simulink model "HoppingModel_Last"  (R2019b)
settings: Solver=FixedStepAuto  StartTime=0.0  StopTime=20  FixedStep=0.005  RelTol=1e-3
undefined symbols (not defined in the file): g, I1, I2, ini_theta1, ini_theta1_d, ini_theta2, ini_theta2_d, ini_w, ini_w_d, ini_x0, ini_x0_d, ini_x1, ini_x1_d, ini_x2, ini_x2_d, ini_y0, ini_y0_d, ini_y1, ini_y1_d, ini_y2, ini_y2_d, M1, M2, r1, r2, theta1_des
libraries: cstblocks x5
settings Model: Creator=fabia  LastModifiedBy=fabia

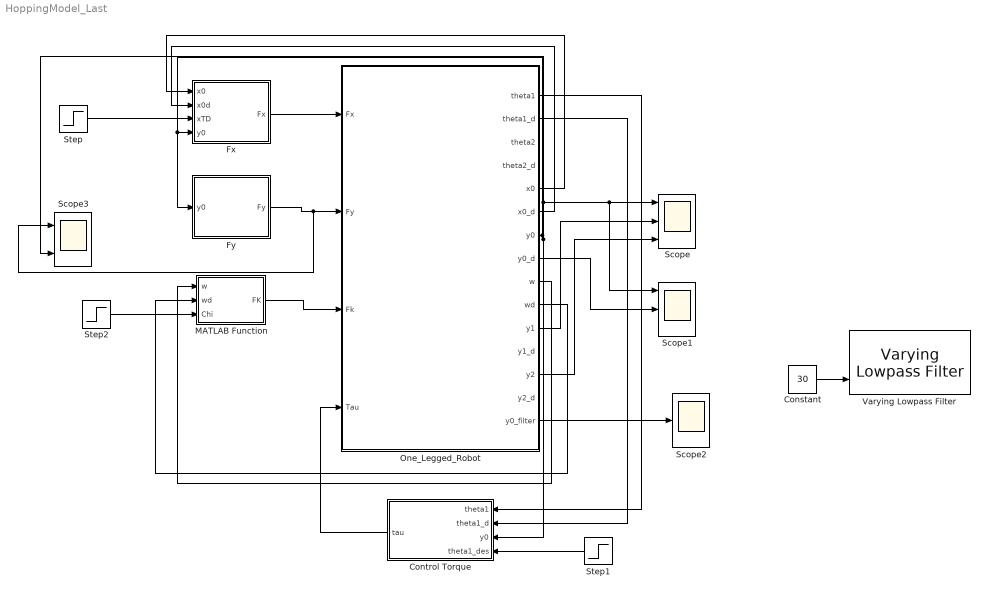
== system HoppingModel_Last ==
  Constant : Constant  Value=30
  Control Torque : MATLAB Function  TreatAsAtomicUnit=on
  Fx : MATLAB Function  TreatAsAtomicUnit=on
  Fy : MATLAB Function  TreatAsAtomicUnit=on
  MATLAB Function : MATLAB Function  TreatAsAtomicUnit=on
  One_Legged_Robot : Subsystem
  Scope : Scope  NumInputPorts=3
  Scope1 : Scope  NumInputPorts=3
  Scope2 : Scope
  Scope3 : Scope  NumInputPorts=2
  Step : Step  Time=0  After=0  SampleTime=0
  Step1 : Step  Time=0  After=theta1_des  SampleTime=0
  Step2 : Step  Time=0  After=0.1  SampleTime=0
  Varying Lowpass Filter : cstblocks/Linear Parameter Varying/Varying Lowpass Filter  N=1
      settings: SourceProductName=Control System Toolbox
  wires:
  Fx/1(Fx) -> One_Legged_Robot/1(Fx)
  One_Legged_Robot/6(x0_d) -> Fx/2(x0d)
  Step/1 -> Fx/3(xTD)
  Step2/1 -> MATLAB Function/3(Chi)
  Control Torque/1(tau) -> One_Legged_Robot/4(Tau)
  One_Legged_Robot/1(theta1) -> Control Torque/1(theta1)
  One_Legged_Robot/2(theta1_d) -> Control Torque/2(theta1_d)
  Step1/1 -> Control Torque/4(theta1_des)
  One_Legged_Robot/11(y1) -> Scope/2
  One_Legged_Robot/13(y2) -> Scope/3
  One_Legged_Robot/7(y0) -> Fy/1(y0), Fx/4(y0), Scope3/2, Scope1/1, Scope/1, Control Torque/3(y0)
  Constant/1 -> Varying Lowpass Filter/2
  One_Legged_Robot/5(x0) -> Fx/1(x0)
  Fy/1(Fy) -> Scope3/1, One_Legged_Robot/2(Fy)
  One_Legged_Robot/9(w) -> MATLAB Function/1(w)
  One_Legged_Robot/10(wd) -> MATLAB Function/2(wd)
  One_Legged_Robot/8(y0_d) -> Scope1/2
  One_Legged_Robot/15(y0_filter) -> Scope2/1
  MATLAB Function/1(FK) -> One_Legged_Robot/3(Fk)

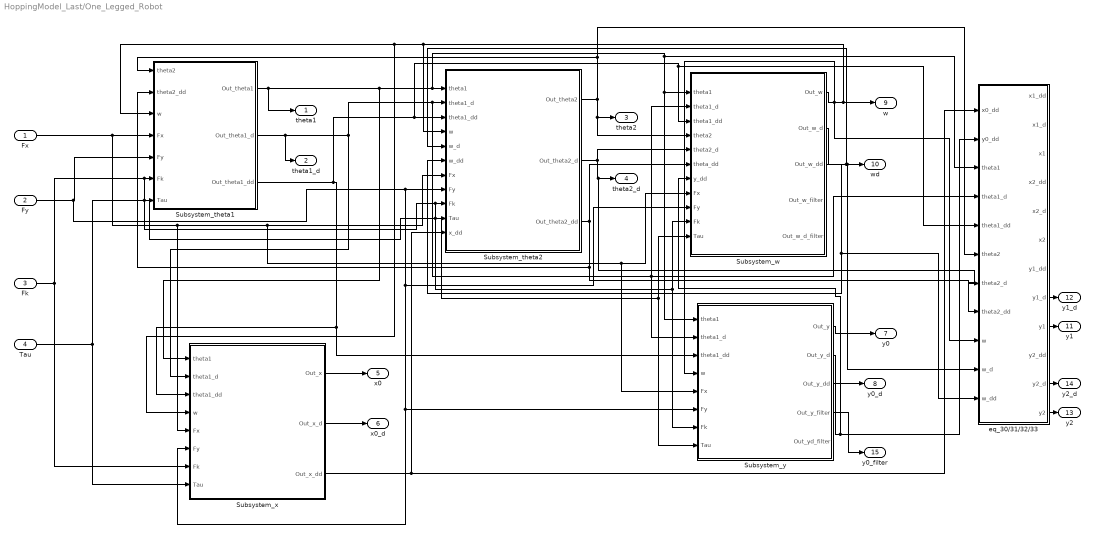
== system HoppingModel_Last/One_Legged_Robot ==
  Fx : Inport
  Fy : Inport  Port=2
  Fk : Inport  Port=3
  Tau : Inport  Port=4
  Subsystem_theta1 : Subsystem
  Subsystem_theta2 : Subsystem
  Subsystem_w : Subsystem
  Subsystem_x : Subsystem
  Subsystem_y : Subsystem
  "eq_30/31/32/33 " : Subsystem
  theta1 : Outport
  theta1_d : Outport  Port=2
  theta2 : Outport  Port=3
  theta2_d : Outport  Port=4
  x0 : Outport  Port=5
  x0_d : Outport  Port=6
  y0 : Outport  Port=7
  y0_d : Outport  Port=8
  w : Outport  Port=9
  wd : Outport  Port=10
  y1 : Outport  Port=11
  y1_d : Outport  Port=12
  y2 : Outport  Port=13
  y2_d : Outport  Port=14
  y0_filter : Outport  Port=15
  wires:
  Subsystem_theta1/1(Out_theta1) -> Subsystem_x/1(theta1), "eq_30/31/32/33 "/3(theta1), Subsystem_y/1(theta1), Subsystem_w/1(theta1), Subsystem_theta2/1(theta1), theta1/1
  Subsystem_theta1/2(Out_theta1_d) -> Subsystem_y/2(theta1_d), "eq_30/31/32/33 "/4(theta1_d), Subsystem_w/2(theta1_d), Subsystem_theta2/2(theta1_d), Subsystem_x/2(theta1_d), theta1_d/1
  Subsystem_x/1(Out_x) -> x0/1
  Subsystem_x/2(Out_x_d) -> x0_d/1
  Subsystem_y/1(Out_y) -> y0/1
  Subsystem_y/2(Out_y_d) -> y0_d/1
  "eq_30/31/32/33 "/9(y1) -> y1/1
  "eq_30/31/32/33 "/8(y1_d) -> y1_d/1
  "eq_30/31/32/33 "/12(y2) -> y2/1
  "eq_30/31/32/33 "/11(y2_d) -> y2_d/1
  Subsystem_w/2(Out_w_d) -> "eq_30/31/32/33 "/10(w_d), wd/1, Subsystem_theta2/5(w_d)
  Subsystem_w/1(Out_w) -> Subsystem_y/4(w), "eq_30/31/32/33 "/9(w), Subsystem_theta2/4(w), Subsystem_x/4(w), Subsystem_theta1/3(w), w/1
  Subsystem_theta2/1(Out_theta2) -> "eq_30/31/32/33 "/6(theta2), Subsystem_theta1/1(theta2), Subsystem_w/4(theta2), theta2/1
  Subsystem_theta2/2(Out_theta2_d) -> Subsystem_w/5(theta2_d), "eq_30/31/32/33 "/7(theta2_d), theta2_d/1
  Subsystem_theta1/3(Out_theta1_dd) -> Subsystem_x/3(theta1_dd), Subsystem_y/3(theta1_dd), "eq_30/31/32/33 "/5(theta1_dd), Subsystem_w/3(theta1_dd), Subsystem_theta2/3(theta1_dd)
  Subsystem_theta2/3(Out_theta2_dd) -> "eq_30/31/32/33 "/8(theta2_dd), Subsystem_theta1/2(theta2_dd), Subsystem_w/6(theta_dd)
  Subsystem_w/3(Out_w_dd) -> "eq_30/31/32/33 "/11(w_dd), Subsystem_theta2/6(w_dd)
  Subsystem_y/3(Out_y_dd) -> "eq_30/31/32/33 "/2(y0_dd), Subsystem_w/7(y_dd)
  Subsystem_x/3(Out_x_dd) -> "eq_30/31/32/33 "/1(x0_dd), Subsystem_theta2/11(x_dd)
  Fx/1 -> Subsystem_x/5(Fx), Subsystem_y/5(Fx), Subsystem_w/8(Fx), Subsystem_theta2/7(Fx), Subsystem_theta1/4(Fx)
  Fy/1 -> Subsystem_w/9(Fy), Subsystem_x/6(Fy), Subsystem_y/6(Fy), Subsystem_theta2/8(Fy), Subsystem_theta1/5(Fy)
  Fk/1 -> Subsystem_x/7(Fk), Subsystem_y/7(Fk), Subsystem_w/10(Fk), Subsystem_theta2/9(Fk), Subsystem_theta1/6(Fk)
  Tau/1 -> Subsystem_x/8(Tau), Subsystem_y/8(Tau), Subsystem_w/11(Tau), Subsystem_theta2/10(Tau), Subsystem_theta1/7(Tau)
  Subsystem_y/4(Out_y_filter) -> y0_filter/1

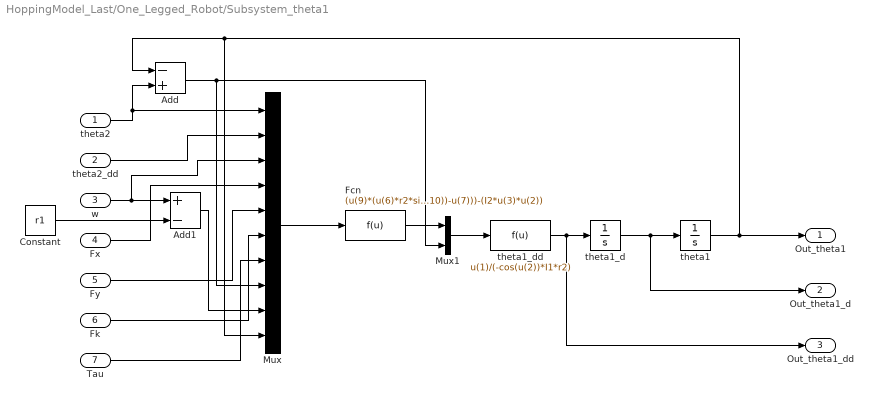
== system HoppingModel_Last/One_Legged_Robot/Subsystem_theta1 ==
  theta2 : Inport
  theta2_dd : Inport  Port=2
  w : Inport  Port=3
  Fx : Inport  Port=4
  Fy : Inport  Port=5
  Fk : Inport  Port=6
  Tau : Inport  Port=7
  Add : Sum  Inputs=-+
  Add1 : Sum  Inputs=+-
  Constant : Constant  Value=r1
  Fcn : Fcn  Expr=(u(9)*(u(6)*r2*sin(u(8))+u(7)))-(r2*cos(u(8))*(r1*u(5)*sin(u(10))-r1*u(4)*cos(u(10))-u(7)))-(I2*u(3)*u(2))
  Mux : Mux  Inputs=10
  Mux1 : Mux  Inputs=2
  theta1 : Integrator  InitialCondition=ini_theta1  LimitOutput=on  UpperSaturationLimit=pi/2  LowerSaturationLimit=-pi/2
  theta1_d : Integrator  InitialCondition=ini_theta1_d  LimitOutput=on  UpperSaturationLimit=pi/2  LowerSaturationLimit=-pi/2
  theta1_dd : Fcn  Expr=u(1)/(-cos(u(2))*I1*r2)
  Out_theta1 : Outport
  Out_theta1_d : Outport  Port=2
  Out_theta1_dd : Outport  Port=3
  wires:
  theta2/1 -> Mux/1, Add/2
  theta1/1 -> Out_theta1/1, Mux/10, Add/1
  w/1 -> Mux/3, Add1/1
  Constant/1 -> Add1/2
  theta2_dd/1 -> Mux/2
  Fx/1 -> Mux/4
  Fy/1 -> Mux/5
  Fk/1 -> Mux/6
  Tau/1 -> Mux/7
  Add/1 -> Mux/8, Mux1/2
  Add1/1 -> Mux/9
  Mux/1 -> Fcn/1
  Fcn/1 -> Mux1/1
  Mux1/1 -> theta1_dd/1
  theta1_dd/1 -> Out_theta1_dd/1, theta1_d/1
  theta1_d/1 -> Out_theta1_d/1, theta1/1

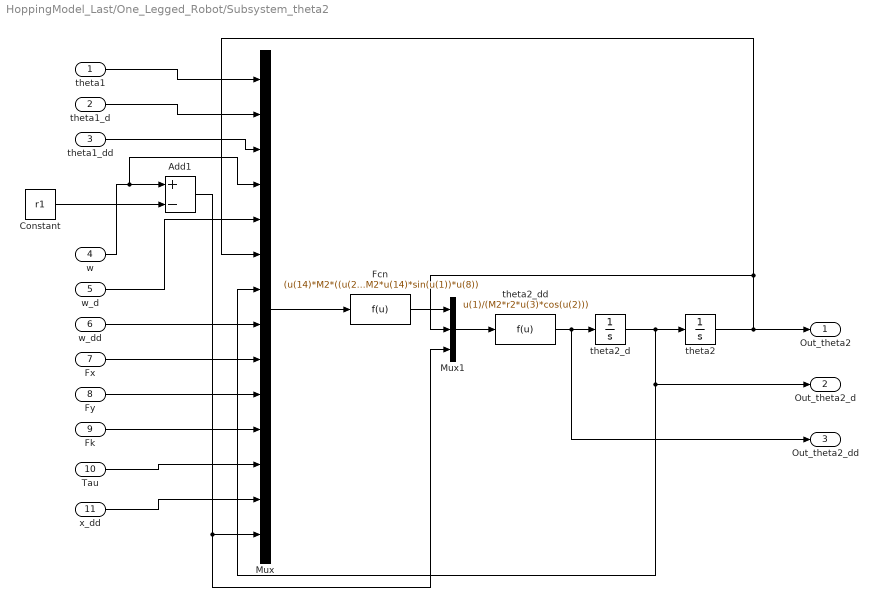
== system HoppingModel_Last/One_Legged_Robot/Subsystem_theta2 ==
  theta1 : Inport
  theta1_d : Inport  Port=2
  theta1_dd : Inport  Port=3
  w : Inport  Port=4
  w_d : Inport  Port=5
  w_dd : Inport  Port=6
  Fx : Inport  Port=7
  Fy : Inport  Port=8
  Fk : Inport  Port=9
  Tau : Inport  Port=10
  x_dd : Inport  Port=11
  Add1 : Sum  Inputs=+-
  Constant : Constant  Value=r1
  Fcn : Fcn  Expr=(u(14)*M2*((u(2)^2)*u(14)*sin(u(1))-2*u(2)*u(5)*cos(u(1))+r2*(u(7)^2)*sin(u(6))+r1*(u(2)^2)*sin(u(1))))-(r1*u(9)*(cos(u(1)))^2)+(cos(u(1))*(r1*u(10)*sin(u(1))-u(12)))+(u(11)*u(14)*sin(u(1)))-(M2*u(14)*u(13))-(cos(u(1))*(M2*u(14)*u(4)+I1)*u(3))-(M2*u(14)*sin(u(1))*u(8))
  Mux : Mux  Inputs=14
  Mux1 : Mux  Inputs=3
  theta2 : Integrator  InitialCondition=ini_theta2
  theta2_d : Integrator  InitialCondition=ini_theta2_d
  theta2_dd : Fcn  Expr=u(1)/(M2*r2*u(3)*cos(u(2)))
  Out_theta2 : Outport
  Out_theta2_d : Outport  Port=2
  Out_theta2_dd : Outport  Port=3
  wires:
  theta2/1 -> Mux1/2, Mux/6, Out_theta2/1
  Fcn/1 -> Mux1/1
  Mux1/1 -> theta2_dd/1
  theta2_dd/1 -> Out_theta2_dd/1, theta2_d/1
  theta2_d/1 -> Mux/7, Out_theta2_d/1, theta2/1
  Constant/1 -> Add1/2
  theta1/1 -> Mux/1
  theta1_d/1 -> Mux/2
  theta1_dd/1 -> Mux/3
  Add1/1 -> Mux1/3, Mux/14
  Mux/1 -> Fcn/1
  w/1 -> Mux/4, Add1/1
  w_d/1 -> Mux/5
  w_dd/1 -> Mux/8
  Fx/1 -> Mux/9
  Fy/1 -> Mux/10
  Fk/1 -> Mux/11
  Tau/1 -> Mux/12
  x_dd/1 -> Mux/13

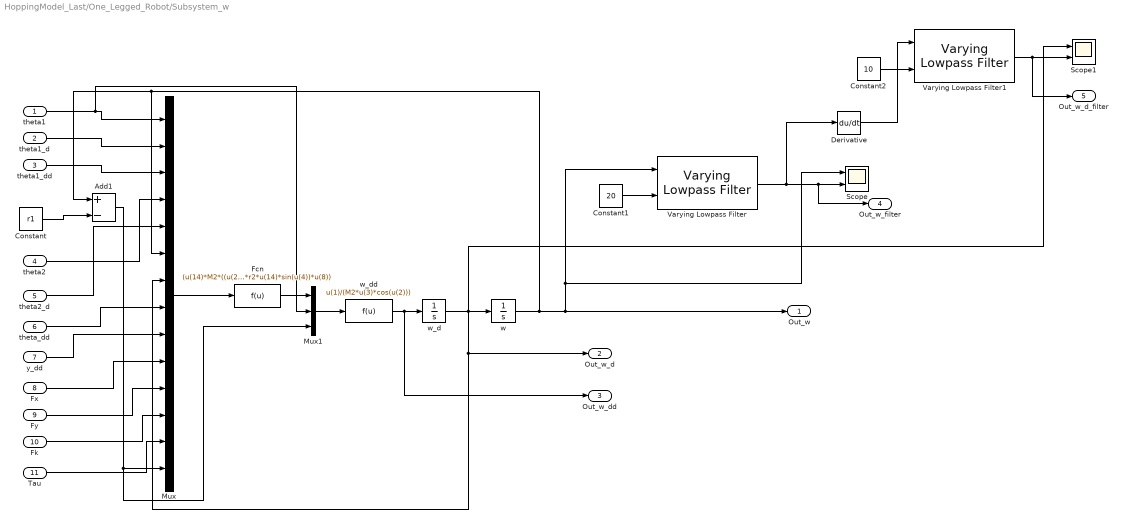
== system HoppingModel_Last/One_Legged_Robot/Subsystem_w ==
  theta1 : Inport
  theta1_d : Inport  Port=2
  theta1_dd : Inport  Port=3
  theta2 : Inport  Port=4
  theta2_d : Inport  Port=5
  theta_dd : Inport  Port=6
  y_dd : Inport  Port=7
  Fx : Inport  Port=8
  Fy : Inport  Port=9
  Fk : Inport  Port=10
  Tau : Inport  Port=11
  Add1 : Sum  Inputs=+-
  Constant : Constant  Value=r1
  Constant1 : Constant  Value=20
  Constant2 : Constant  Value=10
  Derivative : Derivative
  Fcn : Fcn  Expr=(u(14)*M2*((u(2)^2)*u(14)*cos(u(1))+2*u(2)*u(7)*sin(u(1))+r2*(u(5)^2)*cos(u(4))+r1*(u(2)^2)*cos(u(1))-g))+(r1*u(10)*cos(u(1))*sin(u(1)))-(sin(u(1))*(r1*u(11)*sin(u(1))-u(13)))+(u(12)*u(14)*cos(u(1)))+(sin(u(1))*(M2*u(14)*u(6)+I1)*u(3))-(M2*u(14)*u(9))+(M2*r2*u(14)*sin(u(4))*u(8))
  Mux : Mux  Inputs=14
  Mux1 : Mux  Inputs=3
  Scope : Scope  NumInputPorts=2
  Scope1 : Scope  NumInputPorts=2
  Varying Lowpass Filter : cstblocks/Linear Parameter Varying/Varying Lowpass Filter  N=1
      settings: SourceProductName=Control System Toolbox
  Varying Lowpass Filter1 : cstblocks/Linear Parameter Varying/Varying Lowpass Filter  N=1
      settings: SourceProductName=Control System Toolbox
  w : Integrator  InitialCondition=ini_w
  w_d : Integrator  InitialCondition=ini_w_d
  w_dd : Fcn  Expr=u(1)/(M2*u(3)*cos(u(2)))
  Out_w : Outport
  Out_w_d : Outport  Port=2
  Out_w_dd : Outport  Port=3
  Out_w_filter : Outport  Port=4
  Out_w_d_filter : Outport  Port=5
  wires:
  Fcn/1 -> Mux1/1
  Mux1/1 -> w_dd/1
  w_dd/1 -> Out_w_dd/1, w_d/1
  w_d/1 -> Scope1/1, Mux/7, Out_w_d/1, w/1
  Constant/1 -> Add1/2
  Mux/1 -> Fcn/1
  Add1/1 -> Mux1/3, Mux/14
  theta1/1 -> Mux1/2, Mux/1
  theta1_d/1 -> Mux/2
  theta1_dd/1 -> Mux/3
  theta2/1 -> Mux/4
  theta2_d/1 -> Mux/5
  theta_dd/1 -> Mux/8
  y_dd/1 -> Mux/9
  Fx/1 -> Mux/10
  Fy/1 -> Mux/11
  Fk/1 -> Mux/12
  Tau/1 -> Mux/13
  Constant1/1 -> Varying Lowpass Filter/2
  w/1 -> Mux/6, Add1/1, Out_w/1, Scope/1, Varying Lowpass Filter/1
  Derivative/1 -> Varying Lowpass Filter1/1
  Constant2/1 -> Varying Lowpass Filter1/2
  Varying Lowpass Filter/1 -> Derivative/1, Out_w_filter/1, Scope/2
  Varying Lowpass Filter1/1 -> Out_w_d_filter/1, Scope1/2

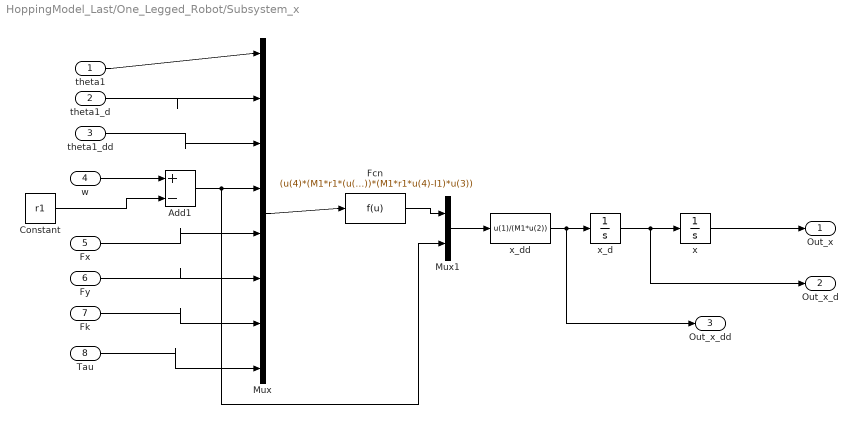
== system HoppingModel_Last/One_Legged_Robot/Subsystem_x ==
  theta1 : Inport
  theta1_d : Inport  Port=2
  theta1_dd : Inport  Port=3
  w : Inport  Port=4
  Fx : Inport  Port=5
  Fy : Inport  Port=6
  Fk : Inport  Port=7
  Tau : Inport  Port=8
  Add1 : Sum  Inputs=+-
  Constant : Constant  Value=r1
  Fcn : Fcn  Expr=(u(4)*(M1*r1*(u(2)^2)*sin(u(1))-u(7)*sin(u(1))+u(5)))-(cos(u(1))*(u(6)*r1*sin(u(1))-u(5)*r1*cos(u(1))-u(8)))-(cos(u(1))*(M1*r1*u(4)-I1)*u(3))
  Mux : Mux  Inputs=8
  Mux1 : Mux  Inputs=2
  x : Integrator  InitialCondition=ini_x0
  x_d : Integrator  InitialCondition=ini_x0_d
  x_dd : Fcn  Expr=u(1)/(M1*u(2))
  Out_x : Outport
  Out_x_d : Outport  Port=2
  Out_x_dd : Outport  Port=3
  wires:
  x/1 -> Out_x/1
  Fcn/1 -> Mux1/1
  Mux1/1 -> x_dd/1
  x_dd/1 -> Out_x_dd/1, x_d/1
  x_d/1 -> Out_x_d/1, x/1
  Constant/1 -> Add1/2
  Mux/1 -> Fcn/1
  w/1 -> Add1/1
  theta1/1 -> Mux/1
  theta1_d/1 -> Mux/2
  theta1_dd/1 -> Mux/3
  Add1/1 -> Mux1/2, Mux/4
  Fx/1 -> Mux/5
  Fy/1 -> Mux/6
  Fk/1 -> Mux/7
  Tau/1 -> Mux/8

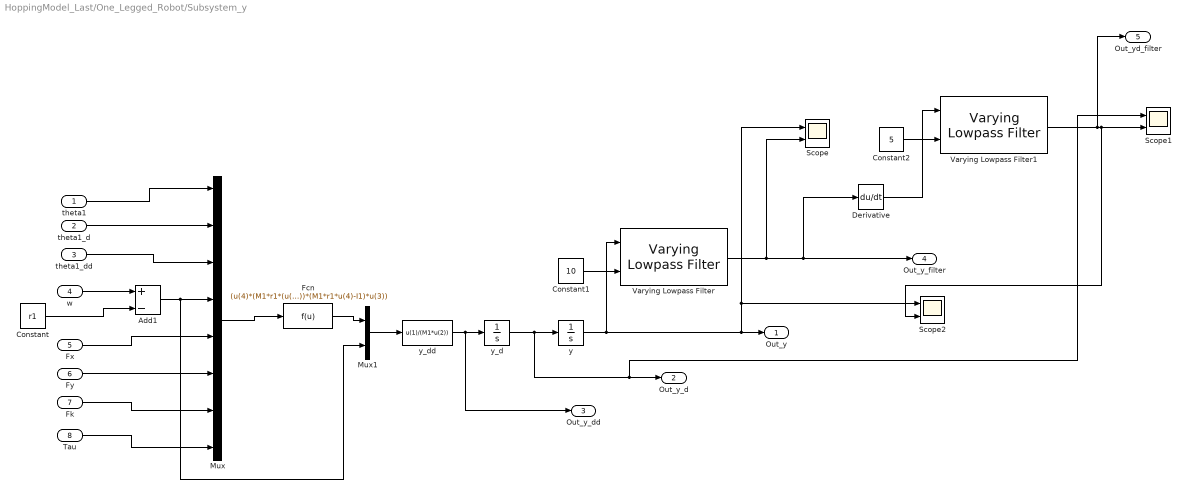
== system HoppingModel_Last/One_Legged_Robot/Subsystem_y ==
  theta1 : Inport
  theta1_d : Inport  Port=2
  theta1_dd : Inport  Port=3
  w : Inport  Port=4
  Fx : Inport  Port=5
  Fy : Inport  Port=6
  Fk : Inport  Port=7
  Tau : Inport  Port=8
  Add1 : Sum  Inputs=+-
  Constant : Constant  Value=r1
  Constant1 : Constant  Value=10
  Constant2 : Constant  Value=5
  Derivative : Derivative
  Fcn : Fcn  Expr=(u(4)*(M1*r1*(u(2)^2)*cos(u(1))-u(7)*cos(u(1))+u(6)-M1*g))-(sin(u(1))*(u(6)*r1*sin(u(1))-u(5)*r1*cos(u(1))-u(8)))+(sin(u(1))*(M1*r1*u(4)-I1)*u(3))
  Mux : Mux  Inputs=8
  Mux1 : Mux  Inputs=2
  Scope : Scope  NumInputPorts=2
  Scope1 : Scope  NumInputPorts=2
  Scope2 : Scope  NumInputPorts=2
  Varying Lowpass Filter : cstblocks/Linear Parameter Varying/Varying Lowpass Filter  N=1
      settings: SourceProductName=Control System Toolbox
  Varying Lowpass Filter1 : cstblocks/Linear Parameter Varying/Varying Lowpass Filter  N=1
      settings: SourceProductName=Control System Toolbox
  y : Integrator  InitialCondition=ini_y0
  y_d : Integrator  InitialCondition=ini_y0_d
  y_dd : Fcn  Expr=u(1)/(M1*u(2))
  Out_y : Outport
  Out_y_d : Outport  Port=2
  Out_y_dd : Outport  Port=3
  Out_y_filter : Outport  Port=4
  Out_yd_filter : Outport  Port=5
  wires:
  Fcn/1 -> Mux1/1
  Mux1/1 -> y_dd/1
  y_dd/1 -> Out_y_dd/1, y_d/1
  y_d/1 -> Scope1/1, Out_y_d/1, y/1
  Constant/1 -> Add1/2
  Mux/1 -> Fcn/1
  w/1 -> Add1/1
  theta1/1 -> Mux/1
  theta1_d/1 -> Mux/2
  theta1_dd/1 -> Mux/3
  Add1/1 -> Mux1/2, Mux/4
  Fx/1 -> Mux/5
  Fy/1 -> Mux/6
  Fk/1 -> Mux/7
  Tau/1 -> Mux/8
  Constant1/1 -> Varying Lowpass Filter/2
  Varying Lowpass Filter/1 -> Derivative/1, Out_y_filter/1, Scope/2
  Constant2/1 -> Varying Lowpass Filter1/2
  Derivative/1 -> Varying Lowpass Filter1/1
  Varying Lowpass Filter1/1 -> Scope1/2, Scope2/2, Out_yd_filter/1
  y/1 -> Scope2/1, Scope/1, Out_y/1, Varying Lowpass Filter/1

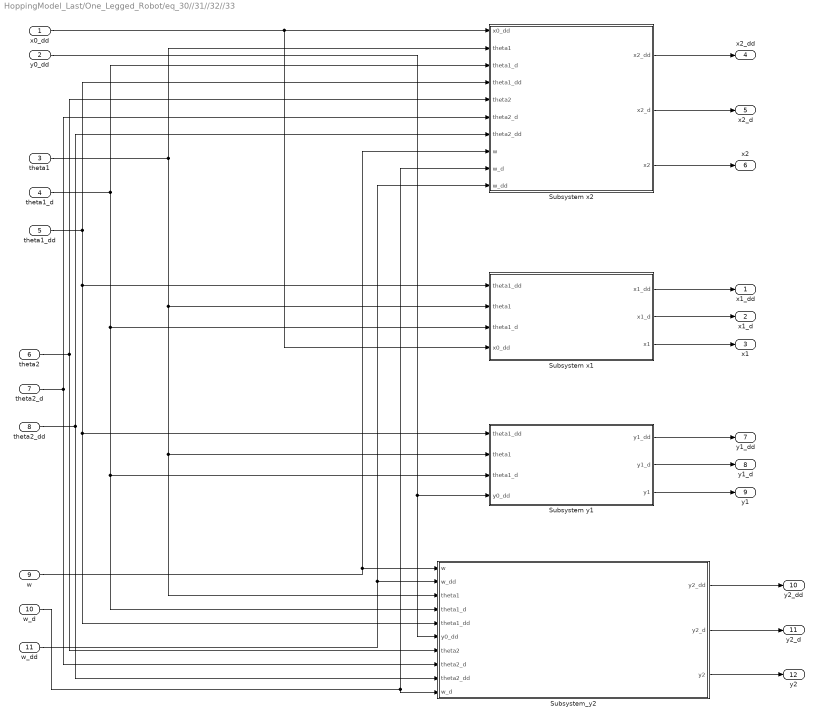
== system HoppingModel_Last/One_Legged_Robot/eq_30//31//32//33  ==
  x0_dd : Inport
  y0_dd : Inport  Port=2
  theta1 : Inport  Port=3
  theta1_d : Inport  Port=4
  theta1_dd : Inport  Port=5
  theta2 : Inport  Port=6
  theta2_d : Inport  Port=7
  theta2_dd : Inport  Port=8
  w : Inport  Port=9
  w_d : Inport  Port=10
  w_dd : Inport  Port=11
  Subsystem x1 : Subsystem
  Subsystem x2 : Subsystem
  Subsystem y1 : Subsystem
  Subsystem_y2 : Subsystem
  x1_dd : Outport
  x1_d : Outport  Port=2
  x1 : Outport  Port=3
  x2_dd : Outport  Port=4
  x2_d : Outport  Port=5
  x2 : Outport  Port=6
  y1_dd : Outport  Port=7
  y1_d : Outport  Port=8
  y1 : Outport  Port=9
  y2_dd : Outport  Port=10
  y2_d : Outport  Port=11
  y2 : Outport  Port=12
  wires:
  Subsystem x1/1(x1_dd) -> x1_dd/1
  Subsystem x1/3(x1) -> x1/1
  x0_dd/1 -> Subsystem x1/4(x0_dd), Subsystem x2/1(x0_dd)
  Subsystem_y2/1(y2_dd) -> y2_dd/1
  theta1_d/1 -> Subsystem_y2/4(theta1_d), Subsystem y1/3(theta1_d), Subsystem x1/3(theta1_d), Subsystem x2/3(theta1_d)
  Subsystem x2/1(x2_dd) -> x2_dd/1
  Subsystem x2/3(x2) -> x2/1
  w_dd/1 -> Subsystem x2/10(w_dd), Subsystem_y2/2(w_dd)
  Subsystem_y2/3(y2) -> y2/1
  theta1/1 -> Subsystem_y2/3(theta1), Subsystem y1/2(theta1), Subsystem x1/2(theta1), Subsystem x2/2(theta1)
  Subsystem x1/2(x1_d) -> x1_d/1
  theta1_dd/1 -> Subsystem_y2/5(theta1_dd), Subsystem y1/1("theta1_dd "), Subsystem x1/1("theta1_dd "), Subsystem x2/4(theta1_dd)
  y0_dd/1 -> Subsystem_y2/6(y0_dd), Subsystem y1/4(y0_dd)
  theta2_dd/1 -> Subsystem x2/7("theta2_dd "), Subsystem_y2/9(theta2_dd)
  w_d/1 -> Subsystem_y2/10(w_d), Subsystem x2/9(w_d)
  Subsystem x2/2(x2_d) -> x2_d/1
  Subsystem y1/3(y1) -> y1/1
  theta2_d/1 -> Subsystem x2/6(theta2_d), Subsystem_y2/8(theta2_d)
  theta2/1 -> Subsystem x2/5(theta2), Subsystem_y2/7(theta2)
  w/1 -> Subsystem x2/8(w), Subsystem_y2/1(w)
  Subsystem y1/2(y1_d) -> y1_d/1
  Subsystem y1/1(y1_dd) -> y1_dd/1
  Subsystem_y2/2(y2_d) -> y2_d/1

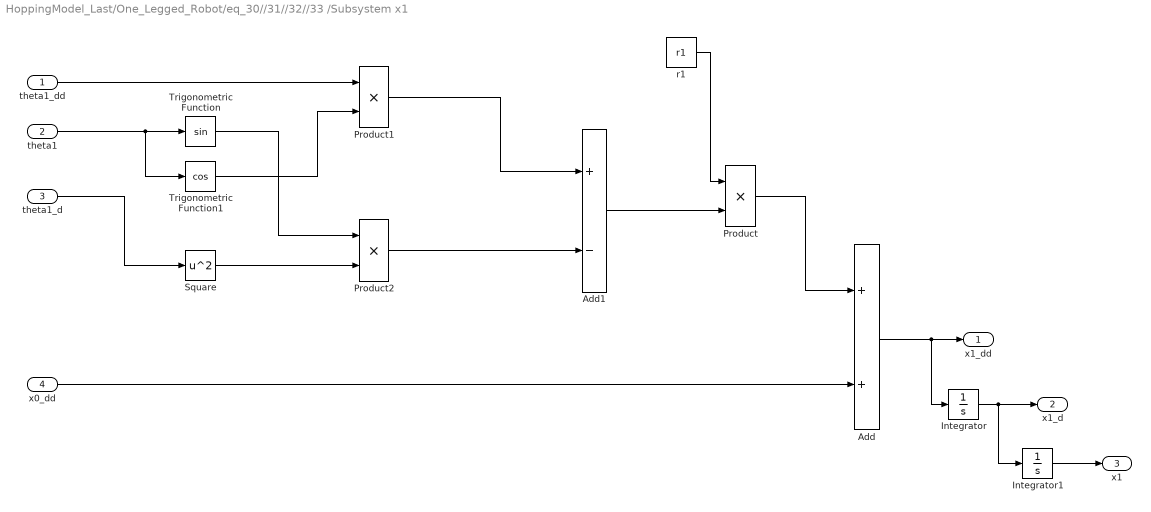
== system HoppingModel_Last/One_Legged_Robot/eq_30//31//32//33 /Subsystem x1 ==
  "theta1_dd " : Inport
  theta1 : Inport  Port=2
  theta1_d : Inport  Port=3
  x0_dd : Inport  Port=4
  Add : Sum
  Add1 : Sum  Inputs=+-
  Integrator : Integrator  InitialCondition=ini_x1_d
  Integrator1 : Integrator  InitialCondition=ini_x1
  Product : Product
  Product1 : Product
  Product2 : Product
  Square : Math  Operator=square  SignedPower=off  SaturateOnIntegerOverflow=on
  Trigonometric Function : Trigonometry
  Trigonometric Function1 : Trigonometry  Operator=cos
  r1 : Constant  Value=r1
  x1_dd : Outport
  x1_d : Outport  Port=2
  x1 : Outport  Port=3
  wires:
  Add1/1 -> Product/2
  Product/1 -> Add/1
  Product2/1 -> Add1/2
  r1/1 -> Product/1
  Trigonometric Function1/1 -> Product1/2
  x0_dd/1 -> Add/2
  theta1_d/1 -> Square/1
  Trigonometric Function/1 -> Product2/1
  Integrator/1 -> x1_d/1, Integrator1/1
  Add/1 -> x1_dd/1, Integrator/1
  Square/1 -> Product2/2
  Product1/1 -> Add1/1
  "theta1_dd "/1 -> Product1/1
  theta1/1 -> Trigonometric Function1/1, Trigonometric Function/1
  Integrator1/1 -> x1/1

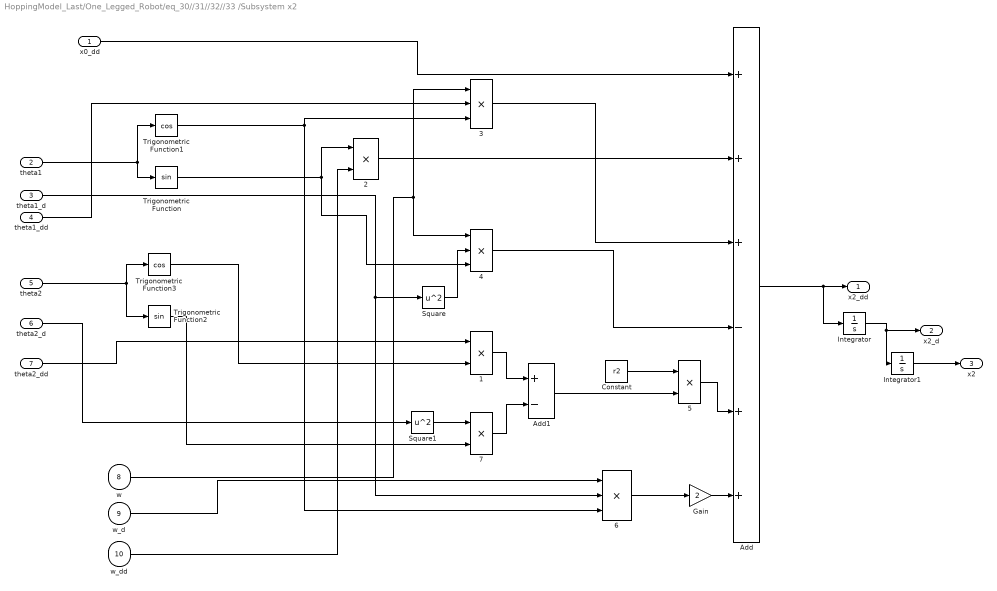
== system HoppingModel_Last/One_Legged_Robot/eq_30//31//32//33 /Subsystem x2 ==
  x0_dd : Inport
  theta1 : Inport  Port=2
  theta1_d : Inport  Port=3
  theta1_dd : Inport  Port=4
  theta2 : Inport  Port=5
  theta2_d : Inport  Port=6
  "theta2_dd " : Inport  Port=7
  w : Inport  Port=8
  w_d : Inport  Port=9
  w_dd : Inport  Port=10
  {1..2,5,7} (4 alike) : Product
  3 : Product  Inputs=3
  4 : Product  Inputs=3
  6 : Product  Inputs=3
  Add : Sum  Inputs=+++-++
  Add1 : Sum  Inputs=+-
  Constant : Constant  Value=r2
  Gain : Gain  Gain=2
  Integrator : Integrator  InitialCondition=ini_x2_d
  Integrator1 : Integrator  InitialCondition=ini_x2
  Square : Math  Operator=square  SignedPower=off  SaturateOnIntegerOverflow=on
  Square1 : Math  Operator=square  SignedPower=off  SaturateOnIntegerOverflow=on
  Trigonometric Function : Trigonometry
  Trigonometric Function1 : Trigonometry  Operator=cos
  Trigonometric Function2 : Trigonometry
  Trigonometric Function3 : Trigonometry  Operator=cos
  x2_dd : Outport
  x2_d : Outport  Port=2
  x2 : Outport  Port=3
  wires:
  7/1 -> Add1/2
  Integrator1/1 -> x2/1
  w_d/1 -> 6/1
  Constant/1 -> 5/1
  Integrator/1 -> x2_d/1, Integrator1/1
  Trigonometric Function1/1 -> 6/3, 3/3
  x0_dd/1 -> Add/1
  Add1/1 -> 5/2
  theta2/1 -> Trigonometric Function3/1, Trigonometric Function2/1
  6/1 -> Gain/1
  4/1 -> Add/4
  Square/1 -> 4/2
  theta1_d/1 -> 6/2, Square/1
  Square1/1 -> 7/1
  w/1 -> 3/1, 4/1
  Add/1 -> x2_dd/1, Integrator/1
  Trigonometric Function2/1 -> 7/2
  Trigonometric Function3/1 -> 1/2
  w_dd/1 -> 2/2
  theta1/1 -> Trigonometric Function1/1, Trigonometric Function/1
  Gain/1 -> Add/6
  Trigonometric Function/1 -> 4/3, 2/1
  theta1_dd/1 -> 3/2
  3/1 -> Add/3
  1/1 -> Add1/1
  2/1 -> Add/2
  5/1 -> Add/5
  "theta2_dd "/1 -> 1/1
  theta2_d/1 -> Square1/1

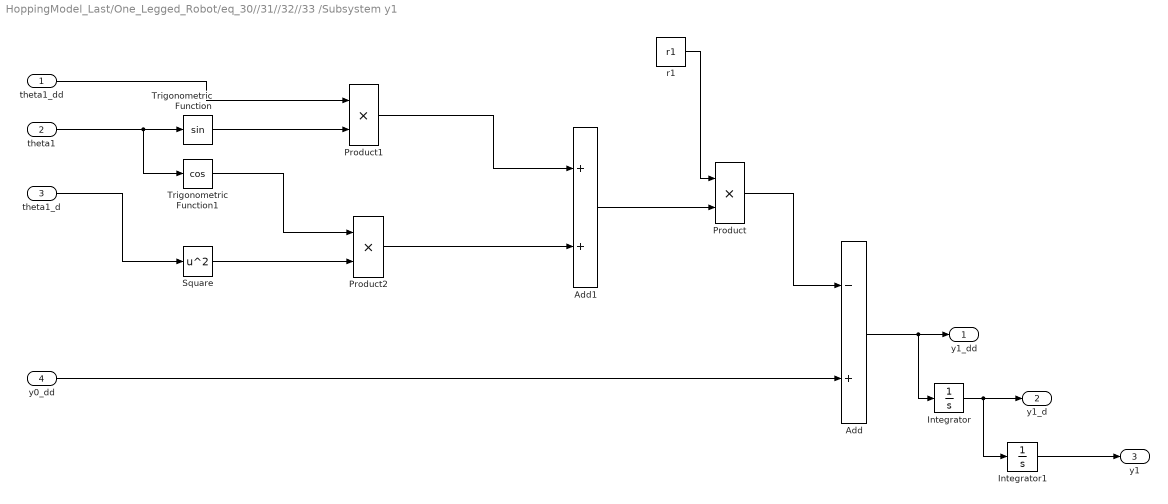
== system HoppingModel_Last/One_Legged_Robot/eq_30//31//32//33 /Subsystem y1 ==
  "theta1_dd " : Inport
  theta1 : Inport  Port=2
  theta1_d : Inport  Port=3
  y0_dd : Inport  Port=4
  Add : Sum  Inputs=-+
  Add1 : Sum
  Integrator : Integrator  InitialCondition=ini_y1_d
  Integrator1 : Integrator  InitialCondition=ini_y1
  Product : Product
  Product1 : Product
  Product2 : Product
  Square : Math  Operator=square  SignedPower=off  SaturateOnIntegerOverflow=on
  Trigonometric Function : Trigonometry
  Trigonometric Function1 : Trigonometry  Operator=cos
  r1 : Constant  Value=r1
  y1_dd : Outport
  y1_d : Outport  Port=2
  y1 : Outport  Port=3
  wires:
  "theta1_dd "/1 -> Product1/1
  Product1/1 -> Add1/1
  y0_dd/1 -> Add/2
  Integrator/1 -> y1_d/1, Integrator1/1
  Add/1 -> y1_dd/1, Integrator/1
  r1/1 -> Product/1
  Integrator1/1 -> y1/1
  theta1/1 -> Trigonometric Function1/1, Trigonometric Function/1
  Square/1 -> Product2/2
  theta1_d/1 -> Square/1
  Product/1 -> Add/1
  Trigonometric Function/1 -> Product1/2
  Product2/1 -> Add1/2
  Add1/1 -> Product/2
  Trigonometric Function1/1 -> Product2/1

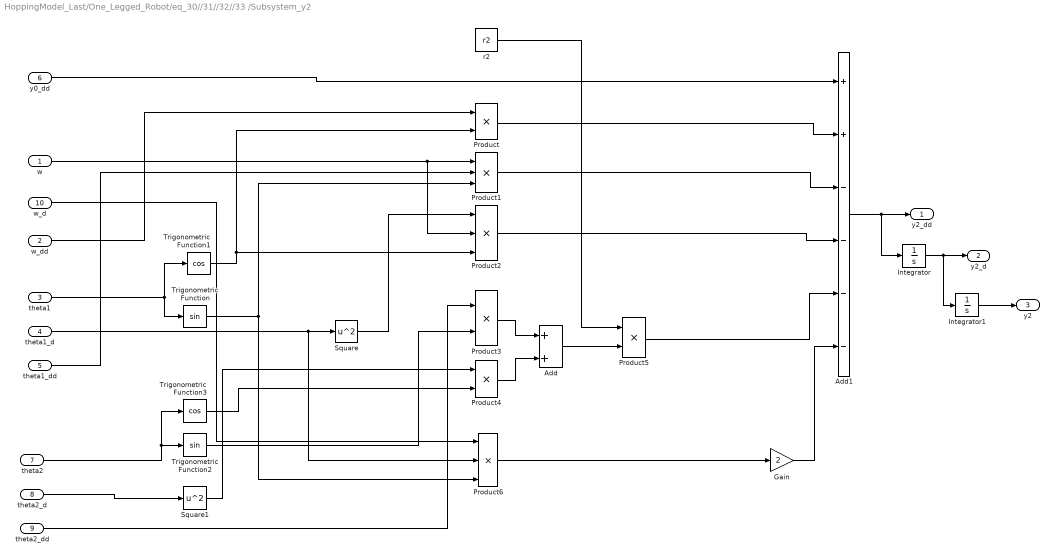
== system HoppingModel_Last/One_Legged_Robot/eq_30//31//32//33 /Subsystem_y2 ==
  w : Inport
  w_dd : Inport  Port=2
  theta1 : Inport  Port=3
  theta1_d : Inport  Port=4
  theta1_dd : Inport  Port=5
  y0_dd : Inport  Port=6
  theta2 : Inport  Port=7
  theta2_d : Inport  Port=8
  theta2_dd : Inport  Port=9
  w_d : Inport  Port=10
  Add : Sum
  Add1 : Sum  Inputs=++----
  Gain : Gain  Gain=2
  Integrator : Integrator  InitialCondition=ini_y2_d
  Integrator1 : Integrator  InitialCondition=ini_y2
  Product{,3..5} (4 alike) : Product
  Product1 : Product  Inputs=3
  Product2 : Product  Inputs=3
  Product6 : Product  Inputs=3
  Square : Math  Operator=square  SignedPower=off  SaturateOnIntegerOverflow=on
  Square1 : Math  Operator=square  SignedPower=off  SaturateOnIntegerOverflow=on
  Trigonometric Function : Trigonometry
  Trigonometric Function1 : Trigonometry  Operator=cos
  Trigonometric Function2 : Trigonometry
  Trigonometric Function3 : Trigonometry  Operator=cos
  r2 : Constant  Value=r2
  y2_dd : Outport
  y2_d : Outport  Port=2
  y2 : Outport  Port=3
  wires:
  r2/1 -> Product5/1
  Product2/1 -> Add1/4
  theta2_d/1 -> Square1/1
  Product5/1 -> Add1/5
  Product1/1 -> Add1/3
  y0_dd/1 -> Add1/1
  Product3/1 -> Add/1
  Product6/1 -> Gain/1
  theta1_d/1 -> Product6/2, Square/1
  Integrator1/1 -> y2/1
  w/1 -> Product2/2, Product1/1
  Trigonometric Function/1 -> Product1/3, Product6/3
  theta1_dd/1 -> Product1/2
  Integrator/1 -> y2_d/1, Integrator1/1
  Product/1 -> Add1/2
  w_d/1 -> Product6/1
  theta1/1 -> Trigonometric Function1/1, Trigonometric Function/1
  w_dd/1 -> Product/1
  Gain/1 -> Add1/6
  Trigonometric Function1/1 -> Product/2, Product2/3
  Square1/1 -> Product4/1
  theta2/1 -> Trigonometric Function3/1, Trigonometric Function2/1
  Add1/1 -> y2_dd/1, Integrator/1
  Product4/1 -> Add/2
  Trigonometric Function2/1 -> Product3/2
  Trigonometric Function3/1 -> Product4/2
  Add/1 -> Product5/2
  Square/1 -> Product2/1
  theta2_dd/1 -> Product3/1

== matlab function HoppingModel_Last/Fx ==
  data: x0 input; Fx output; x0d input; xTD input; y0 input
function Fx = fcn(x0,x0d,xTD,y0)
KG=10^4; % [Nt/m]
BG=75; % [Nt-s/m]
if y0<0
   Fx = -KG*(x0-xTD)-(BG*x0d);
else
   Fx=0;
end

== matlab function HoppingModel_Last/Fy ==
  data: Fy output; y0 input
function Fy = fcn(y0)
KG=10^4; % [Nt/m]
BG=75; % [Nt-s/m]
if y0<0
   Fy = (-KG*y0)-(BG*y0);
else
    Fy=0;
end

== matlab function HoppingModel_Last/MATLAB Function ==
  data: w input; FK output; wd input; Chi input
function FK = fcn(w,wd,Chi)
k0=1; % [m]
KL=10^3; % [Nt/m]

KL2=10^5; % [Nt/m]
BL2=125; % [Nt-s/m]
if (k0-w+Chi)>0
   FK = KL*(k0-w+Chi);
else
    FK=KL2*(k0-w+Chi)-(BL2*wd);
end

== matlab function HoppingModel_Last/Control Torque ==
  data: theta1 input; theta1_d input; y0 input; tau output; theta1_des input
function tau = fcn(theta1,theta1_d,y0, theta1_des)

if y0<=0
    Kp=1800; %[Nt-m/rad]
    Kv=200; %[Nt-m-s/rad]
else
    Kp=1200; %[Nt-m/rad]
    Kv=60; %[Nt-m-s/rad]
end
tau=Kp*(theta1-theta1_des)+Kv*(theta1_d);
